simulink model "motor"  (Simulink 8.7)
settings: Solver=FixedStepAuto  StartTime=0.0  StopTime=2  FixedStep=0.015  RelTol=1e-3
values from neighbouring files (symbols this model uses):
  b = 0.03475    [loadvar.m]
  J = 0.068    [loadvar.m]
  K = 3.475    [loadvar.m]
  L = 0.055    [loadvar.m]
  R = reshape(PARAMS(13:21), 1, 9)    [ANFIS.m]    (also in loadvar.m = 7.56)
settings Model: Creator=maen  LastModifiedBy=smit
settings DataIOCC: SignalLoggingSaveFormat=ModelDataLogs
settings OptimizationCC: ExpressionDepthLimit=2147483647
settings DebuggingCC: SolverPrmCheckMsg=warning  FcnCallInpInsideContextMsg=UseLocalSettings  StateNameClashWarn=warning
settings GRTTargetCC: CombineOutputUpdateFcns=off  GRTInterface=on
settings ConfigComp: CovSFcnEnable=off

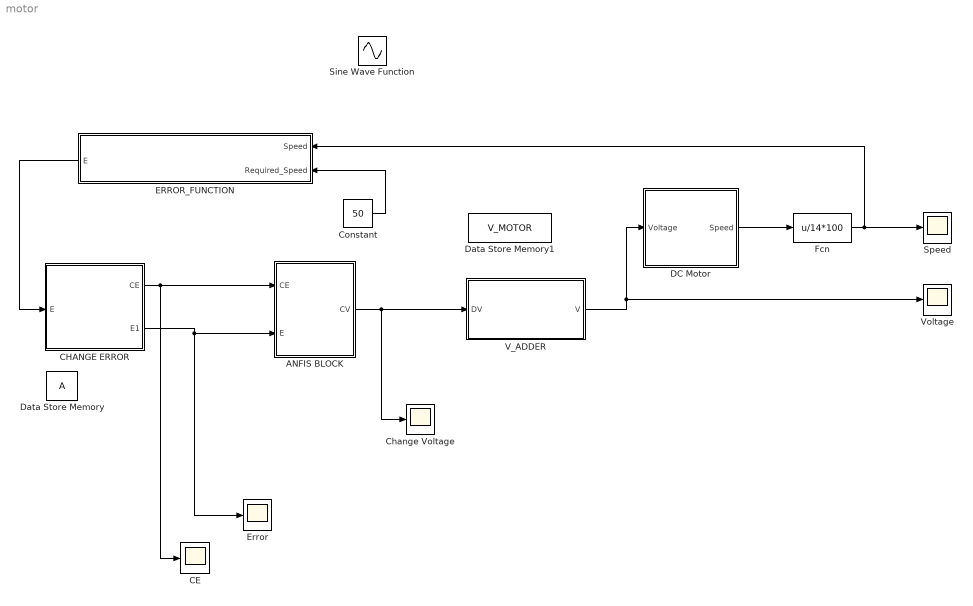
== system motor ==
  ANFIS BLOCK : MATLAB Function  TreatAsAtomicUnit=on
  CE : Scope
  CHANGE ERROR : MATLAB Function  TreatAsAtomicUnit=on
  Change Voltage : Scope
  Constant : Constant  Value=50
  DC Motor : Subsystem
  Data Store Memory : DataStoreMemory  ReadBeforeWriteMsg=warning  WriteAfterWriteMsg=warning  WriteAfterReadMsg=warning  ShowAdditionalParam=off  OutMin=-100  OutMax=100  OutDataTypeStr=double
  Data Store Memory1 : DataStoreMemory  DataStoreName=V_MOTOR  ReadBeforeWriteMsg=warning  WriteAfterWriteMsg=warning  WriteAfterReadMsg=warning  ShowAdditionalParam=off  OutMin=0  OutMax=50  OutDataTypeStr=double
  ERROR_FUNCTION : MATLAB Function  TreatAsAtomicUnit=on
  Error : Scope
  Fcn : Fcn  Expr=u/14*100
  Sine Wave Function : Sin  Amplitude=20  Bias=20  Frequency=5  SampleTime=0
  Speed : Scope
  "V_ADDER " : MATLAB Function  TreatAsAtomicUnit=on
  Voltage : Scope
  wires:
  ANFIS BLOCK/1(CV) -> Change Voltage/1, "V_ADDER "/1(DV)
  DC Motor/1(" Speed") -> Fcn/1
  ERROR_FUNCTION/1(E) -> CHANGE ERROR/1(E)
  CHANGE ERROR/2(E1) -> Error/1, ANFIS BLOCK/2(E)
  "V_ADDER "/1(V) -> DC Motor/1(Voltage), Voltage/1
  Fcn/1 -> Speed/1, ERROR_FUNCTION/1(Speed)
  CHANGE ERROR/1(CE) -> ANFIS BLOCK/1(CE), CE/1
  Constant/1 -> ERROR_FUNCTION/2(Required_Speed)

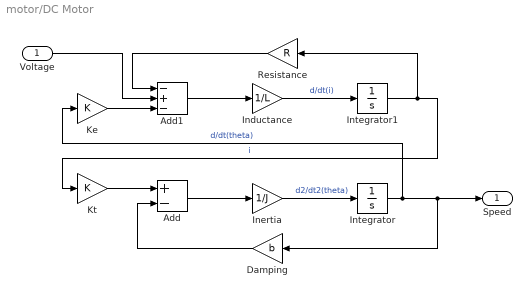
== system motor/DC Motor ==
  Voltage : Inport
  Add : Sum  Inputs=+-
  Add1 : Sum  Inputs=-+-
  Damping : Gain  Gain=b
  Inductance : Gain  Gain=1/L
  Inertia : Gain  Gain=1/J
  Integrator : Integrator
  Integrator1 : Integrator
  Ke : Gain  Gain=K
  Kt : Gain  Gain=K
  Resistance : Gain  Gain=R
  " Speed" : Outport
  wires:
  Integrator1/1 -> Kt/1, Resistance/1  "i"
  Inductance/1 -> Integrator1/1  "d/dt(i)"
  Inertia/1 -> Integrator/1  "d2/dt2(theta)"
  Integrator/1 -> Ke/1, Damping/1, " Speed"/1  "d/dt(theta)"
  Add1/1 -> Inductance/1
  Add/1 -> Inertia/1
  Damping/1 -> Add/2
  Kt/1 -> Add/1
  Resistance/1 -> Add1/1
  Ke/1 -> Add1/3
  Voltage/1 -> Add1/2

== matlab function ERROR_FUNCTION ==
  data: Speed input double; E output double; Required_Speed input double
function E = ERROR_FUNCTION(Speed, Required_Speed)
%#codegen
%pause(0.5);
E = Speed - Required_Speed;

== matlab function ANFIS BLOCK ==
  data: CE input double; E input double; CV output double; A data_store_memory double; V_MOTOR data_store_memory double
function CV =  ANFIS (CE,E)

    %PARAMS= [-1,0,1,-0.5,0,0.5,10,10,10,10,10,10,1,1,0,1,0,-1,0,-1,-1]; 
    PARAMS = [15.84213819	-6.380982431	-1.938824371	-0.303512632	-0.054475133	-0.305344507	22.82157449	23.06081168	21.68859709	2.885971783	2.270890765	2.818305697	-0.663303545	-1.705317671	-0.598665618	2.074496666	1.566314559	-0.613835592	3.026042501	-1.313300156	-2.684444774];

    
    PARAMS  = PARAMS';
    GAUSS_MYU = reshape(PARAMS(1:6), 3, 2)';
    GAUSS_SIG = reshape(PARAMS(7:12), 3, 2)';
    R         = reshape(PARAMS(13:21), 1, 9);
    
    MEMBERSHIP= gaussian(E,CE,GAUSS_MYU,GAUSS_SIG);
    W = zeros(1,9);
    c = 1;
    for i = 1:3
        for j = 1:3
            W(c) = MEMBERSHIP(1,i)*MEMBERSHIP(2,j);
            c = c+1;
        end
    end 
    
    W = W./sum(W);
    
    W1 = W.*R;
    CV = sum(W1);  
    CV = min(5, CV);
    CV = max(-5,CV);
end

function OUT = gaussian(E,CE,GAUSS_MYU,GAUSS_SIG)
    
    OUT      = zeros(2,3);  
    OUT(1,:) = ((GAUSS_MYU(1,:) - E).^2)./(GAUSS_SIG(1,:).^2) ;
    OUT(2,:) = ((GAUSS_MYU(2,:) - CE).^2)./(GAUSS_SIG(2,:).^2); 
    OUT      =  exp(-OUT);
  
end

== matlab function CHANGE ERROR ==
  data: CE output double; E input double; E1 output double; A data_store_memory double
function [CE,E1] = ChangeError(E)
    global A;
    if (A == 0)
        CE = 0;
    else
        CE=(E-A);
    end
    E1=E;
    A=E;
    CE = min(5,CE);
    CE = max(-5,CE);
end

== matlab function V_ADDER  ==
  data: DV input double; V output double; V_MOTOR data_store_memory double
function V = V_ADDER(DV)
    %#codegen
    global V_MOTOR;
    %if(PULSE)
        V_MOTOR = V_MOTOR + DV;
        V_MOTOR = min(50,V_MOTOR);
        V_MOTOR = max(0,V_MOTOR);
    %end
    V= V_MOTOR;
end
